simulink model "lqgf"  (R2016b)
settings: Solver=VariableStepAuto  StartTime=0.0  StopTime=5  RelTol=1e-3
values from neighbouring files (symbols this model uses):
  A = [-Ra1/La1     0            -Kb1/(r*La1)          -Kb1*l/(2*r*La1) ... (first row only)    [lqgfin.m]
  B = [1/La1 0 ... (first row only)    [lqgfin.m]
  C = [0    0    1/r  l/(2*r) ... (first row only)    [lqgfin.m]
  Cx = [0 0 1 0 0 0;0 0 0 1 0 0;0 0 0 0 1 0; 0 0 0 0 0 1]    [lqgfin.m]
  Cy = [1 0 0 0 0 0;0 1 0 0 0 0]    [lqgfin.m]
  D = [0 0 ... (first row only)    [lqgfin.m]
undefined symbols (not defined in the file or in its folder): An, Bn, Cn, Dn, K_lqi
settings Model: Creator=Hamza  LastModifiedBy=Hamza

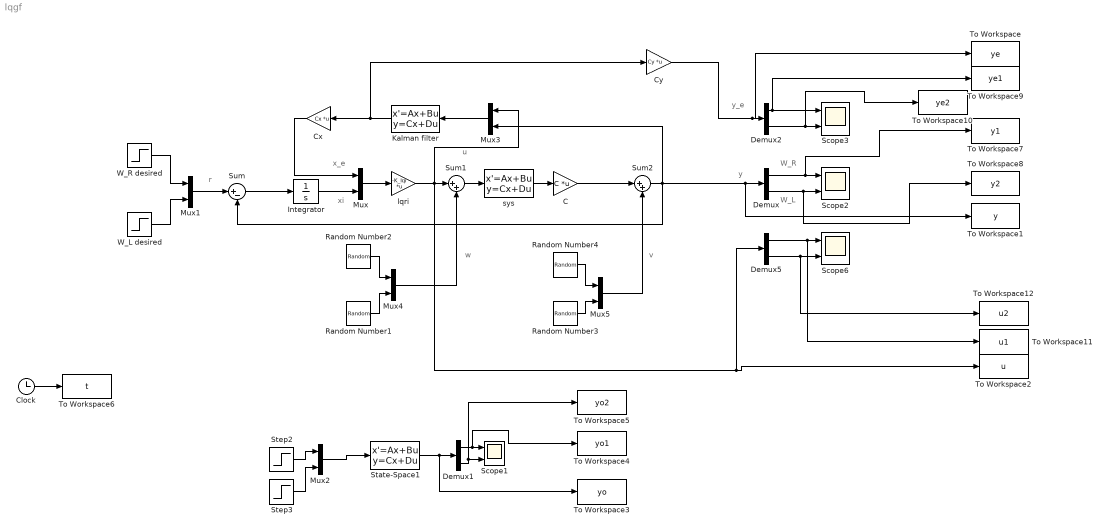
== system lqgf ==
  note: W_R
  note: r
  note: y_e
  note: xi
  note: x_e
  note: u
  note: y
  note: W_L
  note: w
  note: v
  "  Cx" : Gain  Gain=Cx  Multiplication=Matrix(K*u)
  " W_R desired " : Step  After=10  SampleTime=0
  C : Gain  Gain=C  Multiplication=Matrix(K*u)
  Clock : Clock
  Cy : Gain  Gain=Cy  Multiplication=Matrix(K*u)
  Demux{,1..2,5} (4 alike) : Demux  Outputs=2
  Integrator : Integrator
  Kalman filter : StateSpace  A=An  B=Bn  C=Cn  D=Dn  X0=0
  Mux{,1..5} (6 alike) : Mux  Inputs=2
  Random Number1 : RandomNumber  Variance=0.1  Seed=40  SampleTime=0.001
  Random Number2 : RandomNumber  Variance=0.1  Seed=25  SampleTime=0.001
  Random Number3 : RandomNumber  Variance=0.1  Seed=30  SampleTime=0.001
  Random Number4 : RandomNumber  Variance=0.1  Seed=20  SampleTime=0.001
  Scope{1..3,6} (4 alike) : Scope  NumInputPorts=2
  State-Space1 : StateSpace  A=A  B=B  C=C  D=D  X0=0
  Step2 : Step  After=10  SampleTime=0
  Step3 : Step  After=10  SampleTime=0
  Sum : Sum  Inputs=|+-
  Sum1 : Sum  Inputs=|++
  Sum2 : Sum  Inputs=|++
  To Workspace : ToWorkspace  VariableName=ye  SampleTime=-1
  To Workspace1 : ToWorkspace  VariableName=y  SampleTime=-1
  To Workspace10 : ToWorkspace  VariableName=ye2  SampleTime=-1
  To Workspace11 : ToWorkspace  VariableName=u1  SampleTime=-1
  To Workspace12 : ToWorkspace  VariableName=u2  SampleTime=-1
  To Workspace2 : ToWorkspace  VariableName=u  SampleTime=-1
  To Workspace3 : ToWorkspace  VariableName=yo  SampleTime=-1
  To Workspace4 : ToWorkspace  VariableName=yo1  SampleTime=-1
  To Workspace5 : ToWorkspace  VariableName=yo2  SampleTime=-1
  To Workspace6 : ToWorkspace  VariableName=t  SampleTime=-1
  To Workspace7 : ToWorkspace  VariableName=y1  SampleTime=-1
  To Workspace8 : ToWorkspace  VariableName=y2  SampleTime=-1
  To Workspace9 : ToWorkspace  VariableName=ye1  SampleTime=-1
  W_L desired : Step  After=10  SampleTime=0
  lqri : Gain  Gain=-K_lqi  Multiplication=Matrix(K*u)
  sys : StateSpace  A=A  B=B  C=eye(4)  D=zeros(4,2)  X0=0
  wires:
  Sum/1 -> Integrator/1
  Integrator/1 -> Mux/2
  sys/1 -> C/1
  Mux/1 -> lqri/1
  W_L desired/1 -> Mux1/2
  " W_R desired "/1 -> Mux1/1
  Mux1/1 -> Sum/1
  Demux/1 -> To Workspace7/1, Scope2/1
  Demux/2 -> To Workspace8/1, Scope2/2
  Step3/1 -> Mux2/2
  Step2/1 -> Mux2/1
  Mux2/1 -> State-Space1/1
  State-Space1/1 -> To Workspace3/1, Demux1/1
  Demux1/1 -> To Workspace4/1, Scope1/1
  Demux1/2 -> To Workspace5/1, Scope1/2
  Mux3/1 -> Kalman filter/1
  Kalman filter/1 -> Cy/1, "  Cx"/1
  Random Number2/1 -> Mux4/1
  Random Number1/1 -> Mux4/2
  Random Number4/1 -> Mux5/1
  Random Number3/1 -> Mux5/2
  Sum2/1 -> Mux3/2, To Workspace1/1, Demux/1, Sum/2
  Demux2/1 -> To Workspace9/1, Scope3/1
  Demux2/2 -> To Workspace10/1, Scope3/2
  Cy/1 -> To Workspace/1, Demux2/1
  Sum1/1 -> sys/1
  Demux5/1 -> To Workspace11/1, Scope6/1
  Demux5/2 -> To Workspace12/1, Scope6/2
  lqri/1 -> Mux3/1, Demux5/1, To Workspace2/1, Sum1/1
  C/1 -> Sum2/1
  Clock/1 -> To Workspace6/1
  Mux4/1 -> Sum1/2
  Mux5/1 -> Sum2/2
  "  Cx"/1 -> Mux/1
